simulink model "non_linear_sys2"  (R2021b)
settings: Solver=FixedStepAuto  StartTime=0.0  StopTime=Time_simulation  FixedStep=0.01  RelTol=1e-3
values from neighbouring files (symbols this model uses):
  IC = [0.0 0.0]    [data.m]    (also in postproc2.m)
  PID_sim = PID.v1    [data.m]    (also in postproc2.m = PID(PID_idx(ii)))
undefined symbols (not defined in the file or in its folder): amp, fr, ref
libraries: slpidlib x2, dsppolyfun x2
settings Model: Creator=Daniele Oranges  LastModifiedBy=Vincenzo

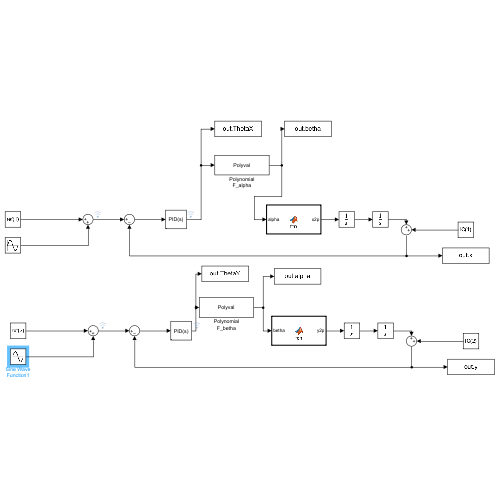
[thumbnail: Simulink's stored preview of the top-level diagram]
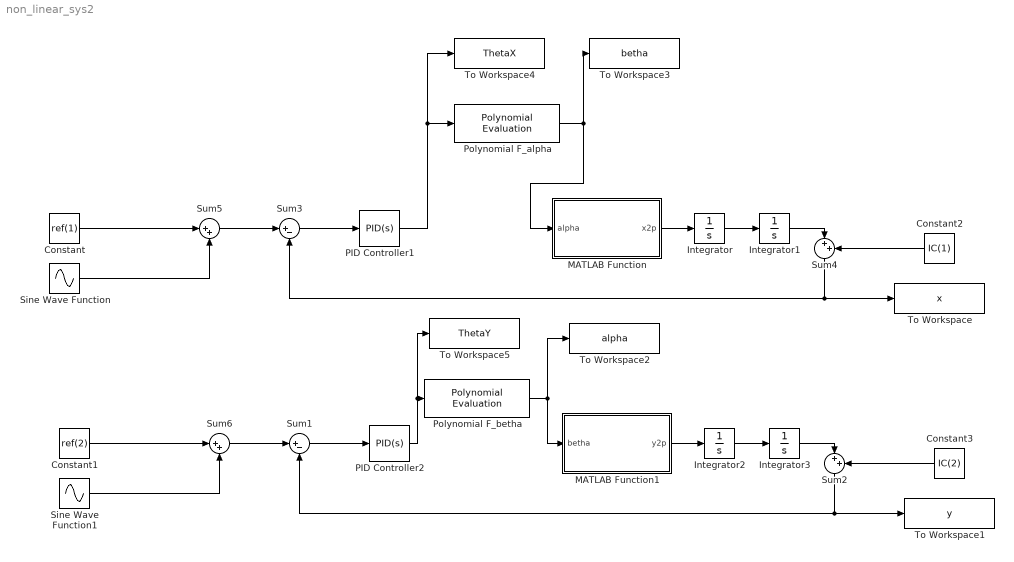
== system non_linear_sys2 ==
  Constant : Constant  Value=ref(1)
  Constant1 : Constant  Value=ref(2)
  Constant2 : Constant  Value=IC(1)
  Constant3 : Constant  Value=IC(2)
  Integrator{,1..3} (4 alike) : Integrator
  MATLAB Function : MATLAB Function  TreatAsAtomicUnit=on
  MATLAB Function1 : MATLAB Function  TreatAsAtomicUnit=on
  PID Controller1 : slpidlib/PID Controller  Controller=PID  Form=Parallel  TimeDomain=Continuous-time  UseExternalTs=off  SampleTime=-1  IntegratorMethod=Forward Euler  FilterMethod=Forward Euler  ControllerParametersSource=internal  P=PID_sim.Kp  I=PID_sim.Ki  D=PID_sim.Kd  UseFilter=on  N=PID_sim.filter  TunerSelectOption=Transfer Function Based (PID Tuner App)  InitialConditionSource=internal  InitialConditionForIntegrator=0  InitialConditionForFilter=0  DifferentiatorICPrevScaledInput=0  ExternalReset=none  TrackingMode=off  Kt=1  LimitOutput=off  SatLimitsSource=internal  UpperSaturationLimit=inf  LowerSaturationLimit=-inf  LinearizeAsGain=on  AntiWindupMode=none  Kb=1  POutMin=[]  POutMax=[]  IOutMin=[]  IOutMax=[]  DOutMin=[]  DOutMax=[]  NOutMin=[]  NOutMax=[]  SumOutMin=[]  SumOutMax=[]  SaturationOutMin=[]  SaturationOutMax=[]  PParamMin=[]  PParamMax=[]  IParamMin=[]  IParamMax=[]  DParamMin=[]  DParamMax=[]  NParamMin=[]  NParamMax=[]  KbParamMin=[]  KbParamMax=[]  KtParamMin=[]  KtParamMax=[]  KbOutMin=[]  KbOutMax=[]  KtOutMin=[]  KtOutMax=[]  IntegratorOutMin=[]  IntegratorOutMax=[]  FilterOutMin=[]  FilterOutMax=[]  SumI1OutMin=[]  SumI1OutMax=[]  SumI2OutMin=[]  SumI2OutMax=[]  SumI3OutMin=[]  SumI3OutMax=[]  SumI4OutMin=[]  SumI4OutMax=[]  SumDOutMin=[]  SumDOutMax=[]  DifferentiatorOutMin=[]  DifferentiatorOutMax=[]  FilterDiffOutCoefMin=[]  FilterDiffOutCoefMax=[]  ReciprocalOutMin=[]  ReciprocalOutMax=[]  SumDenOutMin=[]  SumDenOutMax=[]  SumNumOutMin=[]  SumNumOutMax=[]  DivideOutMin=[]  DivideOutMax=[]  UdiffTsProdOutMin=[]  UdiffTsProdOutMax=[]  NTsProdOutMin=[]  NTsProdOutMax=[]  UintegralTsProdOutMin=[]  UintegralTsProdOutMax=[]  UngainTsProdOutMin=[]  UngainTsProdOutMax=[]  IntegratorContinuousStateAttributes=''  IntegratorStateMustResolveToSignalObject=off  IntegratorRTWStateStorageClass=Auto  FilterContinuousStateAttributes=''  FilterStateMustResolveToSignalObject=off  FilterRTWStateStorageClass=Auto  ParallelPVariant=InternalParameters  IdealPVariant=Disabled  IVariant=InternalParameters  DVariant=InternalParameters  IntegratorVariant=Continuous  SatVariant=Disabled  AWVariant=Passthrough  PCopyVariant=Disabled  TRVariant=Disabled  FdbkBlocksVariant=Forward  IdealPFdbkVariant=Disabled  SatFdbkVariant=Disabled  DerivativeFilterVariant=ContFilter  NVariant=InternalParameters  NCopyVariant=Disabled  FilterICVariant=InternalICsFilter  IntegratorICVariant=InternalICs  ExternalResetVariant=Disabled  TRSumVariant=Passthrough  SumFdbkVariant=Disabled  SumVariant=Sum_PID  TsampFilterVariant=InternalTs  TsampNgainVariant=Passthrough  TsampIntegralVariant=Passthrough  ExternalSaturationOutDataTypeStr=Inherit: Same as second input
  PID Controller2 : slpidlib/PID Controller  Controller=PID  Form=Parallel  TimeDomain=Continuous-time  UseExternalTs=off  SampleTime=-1  IntegratorMethod=Forward Euler  FilterMethod=Forward Euler  ControllerParametersSource=internal  P=PID_sim.Kp  I=PID_sim.Ki  D=PID_sim.Kd  UseFilter=on  N=PID_sim.filter  TunerSelectOption=Transfer Function Based (PID Tuner App)  InitialConditionSource=internal  InitialConditionForIntegrator=0  InitialConditionForFilter=0  DifferentiatorICPrevScaledInput=0  ExternalReset=none  TrackingMode=off  Kt=1  LimitOutput=off  SatLimitsSource=internal  UpperSaturationLimit=inf  LowerSaturationLimit=-inf  LinearizeAsGain=on  AntiWindupMode=none  Kb=1  POutMin=[]  POutMax=[]  IOutMin=[]  IOutMax=[]  DOutMin=[]  DOutMax=[]  NOutMin=[]  NOutMax=[]  SumOutMin=[]  SumOutMax=[]  SaturationOutMin=[]  SaturationOutMax=[]  PParamMin=[]  PParamMax=[]  IParamMin=[]  IParamMax=[]  DParamMin=[]  DParamMax=[]  NParamMin=[]  NParamMax=[]  KbParamMin=[]  KbParamMax=[]  KtParamMin=[]  KtParamMax=[]  KbOutMin=[]  KbOutMax=[]  KtOutMin=[]  KtOutMax=[]  IntegratorOutMin=[]  IntegratorOutMax=[]  FilterOutMin=[]  FilterOutMax=[]  SumI1OutMin=[]  SumI1OutMax=[]  SumI2OutMin=[]  SumI2OutMax=[]  SumI3OutMin=[]  SumI3OutMax=[]  SumI4OutMin=[]  SumI4OutMax=[]  SumDOutMin=[]  SumDOutMax=[]  DifferentiatorOutMin=[]  DifferentiatorOutMax=[]  FilterDiffOutCoefMin=[]  FilterDiffOutCoefMax=[]  ReciprocalOutMin=[]  ReciprocalOutMax=[]  SumDenOutMin=[]  SumDenOutMax=[]  SumNumOutMin=[]  SumNumOutMax=[]  DivideOutMin=[]  DivideOutMax=[]  UdiffTsProdOutMin=[]  UdiffTsProdOutMax=[]  NTsProdOutMin=[]  NTsProdOutMax=[]  UintegralTsProdOutMin=[]  UintegralTsProdOutMax=[]  UngainTsProdOutMin=[]  UngainTsProdOutMax=[]  IntegratorContinuousStateAttributes=''  IntegratorStateMustResolveToSignalObject=off  IntegratorRTWStateStorageClass=Auto  FilterContinuousStateAttributes=''  FilterStateMustResolveToSignalObject=off  FilterRTWStateStorageClass=Auto  ParallelPVariant=InternalParameters  IdealPVariant=Disabled  IVariant=InternalParameters  DVariant=InternalParameters  IntegratorVariant=Continuous  SatVariant=Disabled  AWVariant=Passthrough  PCopyVariant=Disabled  TRVariant=Disabled  FdbkBlocksVariant=Forward  IdealPFdbkVariant=Disabled  SatFdbkVariant=Disabled  DerivativeFilterVariant=ContFilter  NVariant=InternalParameters  NCopyVariant=Disabled  FilterICVariant=InternalICsFilter  IntegratorICVariant=InternalICs  ExternalResetVariant=Disabled  TRSumVariant=Passthrough  SumFdbkVariant=Disabled  SumVariant=Sum_PID  TsampFilterVariant=InternalTs  TsampNgainVariant=Passthrough  TsampIntegralVariant=Passthrough  ExternalSaturationOutDataTypeStr=Inherit: Same as second input
  Polynomial F_alpha : dsppolyfun/Polynomial Evaluation  useConstCoeffs=on  constCoeffs=[-0.0038 -0.0240 -0.0050 0.1698 0]
      settings: SourceProductBaseCode=DS
  Polynomial F_betha : dsppolyfun/Polynomial Evaluation  useConstCoeffs=on  constCoeffs=[-0.0030 -0.0189 -0.0031 0.1318 0.0]
      settings: SourceProductBaseCode=DS
  Sine Wave Function : Sin  Amplitude=amp(1)  Frequency=2*pi*fr(1)  SampleTime=0
  Sine Wave Function1 : Sin  Amplitude=amp(2)  Frequency=2*pi*fr(2)  Phase=pi/2  SampleTime=0
  Sum1 : Sum  Inputs=|+-
  Sum{2,4..6} (4 alike) : Sum  Inputs=|++
  Sum3 : Sum  Inputs=|+-
  To Workspace : ToWorkspace  VariableName=x  SaveFormat=Timeseries  SampleTime=-1
  To Workspace1 : ToWorkspace  VariableName=y  SaveFormat=Timeseries  SampleTime=-1
  To Workspace2 : ToWorkspace  VariableName=alpha  SaveFormat=Timeseries  SampleTime=-1
  To Workspace3 : ToWorkspace  VariableName=betha  SaveFormat=Timeseries  SampleTime=-1
  To Workspace4 : ToWorkspace  VariableName=ThetaX  SaveFormat=Timeseries  SampleTime=-1
  To Workspace5 : ToWorkspace  VariableName=ThetaY  SaveFormat=Timeseries  SampleTime=-1
  wires:
  Sum3/1 -> PID Controller1/1
  Integrator/1 -> Integrator1/1
  MATLAB Function/1(x2p) -> Integrator/1
  Sum1/1 -> PID Controller2/1
  MATLAB Function1/1(y2p) -> Integrator2/1
  Integrator2/1 -> Integrator3/1
  Sum4/1 -> To Workspace/1, Sum3/2
  Constant3/1 -> Sum2/2
  Constant2/1 -> Sum4/2
  Sum2/1 -> Sum1/2, To Workspace1/1
  Integrator1/1 -> Sum4/1
  Integrator3/1 -> Sum2/1
  PID Controller1/1 -> To Workspace4/1, Polynomial F_alpha/1
  Polynomial F_alpha/1 -> MATLAB Function/1(alpha), To Workspace3/1
  PID Controller2/1 -> Polynomial F_betha/1, To Workspace5/1
  Polynomial F_betha/1 -> MATLAB Function1/1(betha), To Workspace2/1
  Sum5/1 -> Sum3/1
  Sine Wave Function/1 -> Sum5/2
  Constant/1 -> Sum5/1
  Sine Wave Function1/1 -> Sum6/2
  Constant1/1 -> Sum6/1
  Sum6/1 -> Sum1/1

== matlab function non_linear_sys2/MATLAB Function ==
  data: alpha input; x2p output
function x2p  = fcn(alpha)
%% Data

g = 9.81;   % gravitational acceleration [m / s^2]

% Dimensions   [m]
Lx = 0.143;                         % joint position in x direction 
Ly = 0.184;                         % joint position in y direction 
Lx_plane=0.15;                        % plane dimension in x direction 
Ly_plane=0.20 ;                       % plane dimension in y direction      
rm = 0.0245;                        % motor arm length 
lm=0.072 ;                          % motor rod length 
pt = 0.005;                          % plane tickness
d=0.021;                            % plane offset

Mot_Osci_Rang=[-80 ,80];    %(deg)   range di oscilazione dei motori                  
% Ball data                 
rb = 0.02;                          % radius of the ball [m]
mb = 0.265;                         % mass of the ball [kg]
Jb = 0.0000416;                     % rotarional inertia of the ball [kg * m^2]
rho_ball = mb/(4/3 * pi * rb^3);    % ball density [Kg/m^3]


x2p = (mb * g * rb^2) / ( mb * rb^2 + Jb ) * sin(alpha);    % x direction transfer function


end

== matlab function non_linear_sys2/MATLAB Function1 ==
  data: betha input; y2p output
function y2p  = fcn(betha)
%% Data

g = 9.81;   % gravitational acceleration [m / s^2]

% Dimensions   [m]
Lx = 0.143;                         % joint position in x direction 
Ly = 0.184;                         % joint position in y direction 
Lx_plane=0.15;                        % plane dimension in x direction 
Ly_plane=0.20 ;                       % plane dimension in y direction      
rm = 0.0245;                        % motor arm length 
lm=0.072 ;                          % motor rod length 
pt = 0.005;                          % plane tickness
d=0.021;                            % plane offset

Mot_Osci_Rang=[-80 ,80];    %(deg)   range di oscilazione dei motori                  
% Ball data                 
rb = 0.02;                          % radius of the ball [m]
mb = 0.265;                         % mass of the ball [kg]
Jb = 0.0000416;                     % rotarional inertia of the ball [kg * m^2]
rho_ball = mb/(4/3 * pi * rb^3);    % ball density [Kg/m^3]


y2p = (mb * g * rb^2) / (mb * rb^2 + Jb) * sin(betha);   % x direction transfer function


end
